simulink model "closedloop"  (R2023a)
settings: Solver=VariableStepAuto  StartTime=0.0  StopTime=21  RelTol=1e-3
values from neighbouring files (symbols this model uses):
  absolute_encoder_counts_per_revolution = 4096    [ELEN90064_Project_Parameters.m]
  init = [theta_m_init; theta_l_init; thetadot_m_init; thetadot_l_init; Ia_init]    [ELEN90064_Project_Parameters.m]
  V_bar = ((T_bar / K_m) + I_noload) * R    [linearised_incremental.m]
  wave_amplitude = deg2rad(15)    [ELEN90064_Project_Parameters.m]
  wave_offset = deg2rad(30)    [ELEN90064_Project_Parameters.m]
  wave_period = 6    [ELEN90064_Project_Parameters.m]
  x2_bar = pi / 6    (= 0.523598775598)    [linearised_incremental.m]    (also in reduced_order.m = deg2rad(30))
undefined symbols (not defined in the file or in its folder): c_a, c_b, sys_a, sys_b
settings Model: Creator=yunzh  LastModifiedBy=yunzh

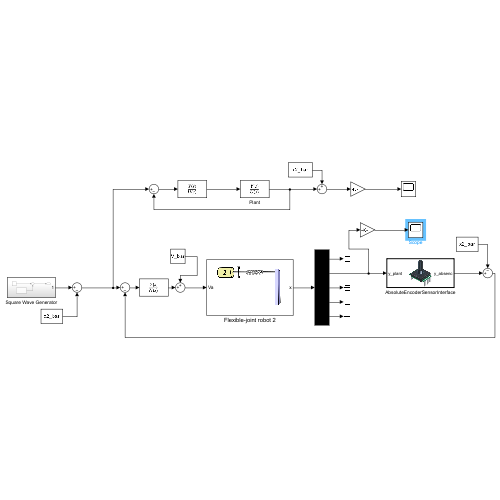
[thumbnail: Simulink's stored preview of the top-level diagram]
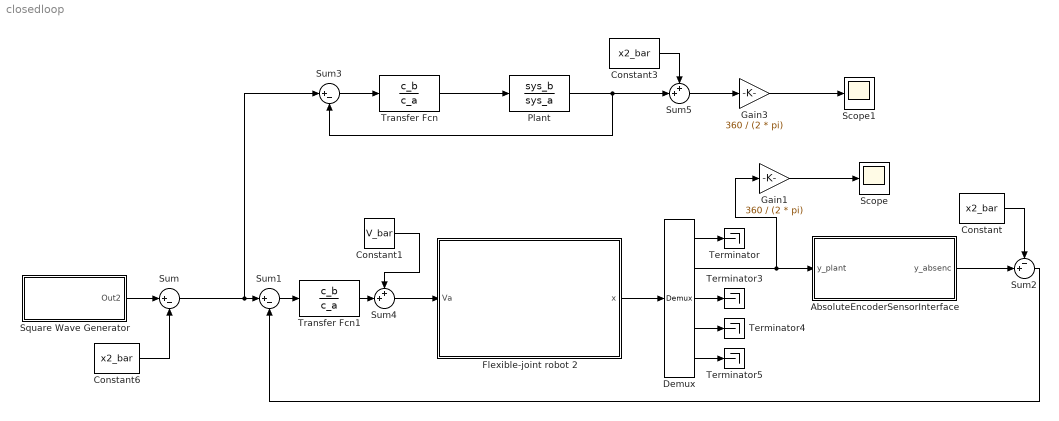
== system closedloop ==
  AbsoluteEncoderSensorInterface : Subsystem  TreatAsAtomicUnit=on
      mask Display: image('$imagefile'); % Use "Edit Image" on toolstrip to change.
  Constant : Constant  Value=x2_bar
  Constant1 : Constant  Value=V_bar
  Constant3 : Constant  Value=x2_bar
  Constant6 : Constant  Value=x2_bar
  Demux : Demux  Outputs=5
  Flexible-joint robot 2 : Subsystem
      mask Display: image('$imagefile'); % Use "Edit Image" on toolstrip to change.
  Gain1 : Gain  Gain=360 / (2 * pi)
  Gain3 : Gain  Gain=360 / (2 * pi)
  Plant : TransferFcn  Numerator=sys_b  Denominator=sys_a
  Scope : Scope
  Scope1 : Scope
  Square Wave Generator : Subsystem
  Sum : Sum  Inputs=|+-
  Sum1 : Sum  Inputs=|+-
  Sum2 : Sum  Inputs=-+|
  Sum3 : Sum  Inputs=|+-
  Sum4 : Sum  Inputs=++|
  Sum5 : Sum  Inputs=++|
  Terminator{,3..5} (4 alike) : Terminator
  Transfer Fcn : TransferFcn  Numerator=c_b  Denominator=c_a
  Transfer Fcn1 : TransferFcn  Numerator=c_b  Denominator=c_a
  wires:
  Flexible-joint robot 2/1(x) -> Demux/1
  Demux/4 -> Terminator4/1
  Demux/5 -> Terminator5/1
  Demux/3 -> Terminator3/1
  Demux/1 -> Terminator/1
  Demux/2 -> AbsoluteEncoderSensorInterface/1(y_plant), Gain1/1
  Sum1/1 -> Transfer Fcn1/1
  Gain1/1 -> Scope/1
  Sum3/1 -> Transfer Fcn/1
  Gain3/1 -> Scope1/1
  Plant/1 -> Sum5/2, Sum3/2
  Constant/1 -> Sum2/1
  Sum2/1 -> Sum1/2
  Transfer Fcn1/1 -> Sum4/2
  Sum4/1 -> Flexible-joint robot 2/1(Va)
  Constant1/1 -> Sum4/1
  Transfer Fcn/1 -> Plant/1
  Sum5/1 -> Gain3/1
  Constant3/1 -> Sum5/1
  Square Wave Generator/1(Out2) -> Sum/1
  Sum/1 -> Sum3/1, Sum1/1
  Constant6/1 -> Sum/2
  AbsoluteEncoderSensorInterface/1(y_absenc) -> Sum2/2

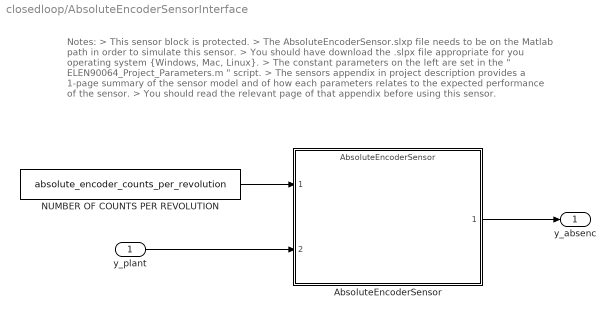
== system closedloop/AbsoluteEncoderSensorInterface ==
  note: Notes:
      | > This sensor block is protected.
      | > The AbsoluteEncoderSensor.slxp file needs to be on the Matlab path in order to simulate this sensor.
      | > You should have download the .slpx file appropriate for you operating system {Windows, Mac, Linux}.
      | > The constant parameters on the left are set in the " ELEN90064_Project_Parameters.m " script.
      | > The sensors appendix in project description provides a 1-page summary of the sensor model and of how each parameters relates to the expected performance of the sensor.
      | > You should read the relevant page of that appendix before using this sensor.
  y_plant : Inport
  AbsoluteEncoderSensor : ModelReference  ModelNameDialog=AbsoluteEncoderSensor.slxp  ModelReferenceVersion=1.16  CopyOfModelProtected=on
  NUMBER OF COUNTS PER REVOLUTION : Constant  Value=absolute_encoder_counts_per_revolution
  y_absenc : Outport
  wires:
  NUMBER OF COUNTS PER REVOLUTION/1 -> AbsoluteEncoderSensor/1
  y_plant/1 -> AbsoluteEncoderSensor/2
  AbsoluteEncoderSensor/1 -> y_absenc/1

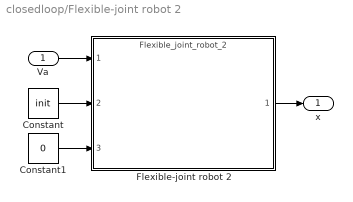
== system closedloop/Flexible-joint robot 2 ==
  Va : Inport
  Constant : Constant  Value=init
  Constant1 : Constant  Value=0
  Flexible-joint robot 2 : ModelReference  ModelNameDialog=Flexible_joint_robot_2  ModelReferenceVersion=1.65  CopyOfModelProtected=on
  x : Outport
  wires:
  Va/1 -> Flexible-joint robot 2/1
  Constant1/1 -> Flexible-joint robot 2/3
  Constant/1 -> Flexible-joint robot 2/2
  Flexible-joint robot 2/1 -> x/1

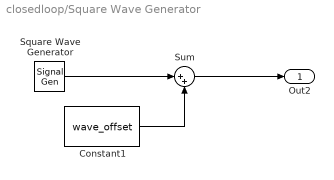
== system closedloop/Square Wave Generator ==
  Constant1 : Constant  Value=wave_offset
  Square Wave Generator : SignalGenerator  WaveForm=square  Amplitude=wave_amplitude  Frequency=1 / wave_period
  Sum : Sum  Inputs=|++
  Out2 : Outport
  wires:
  Square Wave Generator/1 -> Sum/1
  Constant1/1 -> Sum/2
  Sum/1 -> Out2/1
